simulink model "whirlybird_sim"  (Simulink 8.3)
settings: Solver=ode45  StartTime=0.0  StopTime=100  RelTol=1e-3
settings Model: Creator=Administrator  LastModifiedBy=jhl48
settings OptimizationCC: ExpressionDepthLimit=2147483647
settings DebuggingCC: FcnCallInpInsideContextMsg=UseLocalSettings

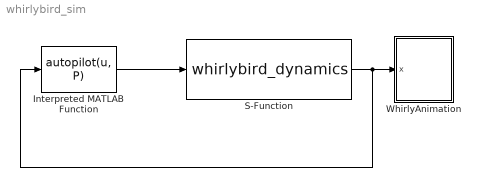
== system whirlybird_sim ==
  Interpreted MATLAB Function : MATLABFcn  MATLABFcn=autopilot(u, P)  OutputDimensions=2
  S-Function : S-Function  FunctionName=whirlybird_dynamics  Parameters=P  EnableBusSupport=off
  WhirlyAnimation : Subsystem
      mask Display: image(imread('tv.jpg'))
  wires:
  S-Function/1 -> Interpreted MATLAB Function/1, WhirlyAnimation/1(x)
  Interpreted MATLAB Function/1 -> S-Function/1

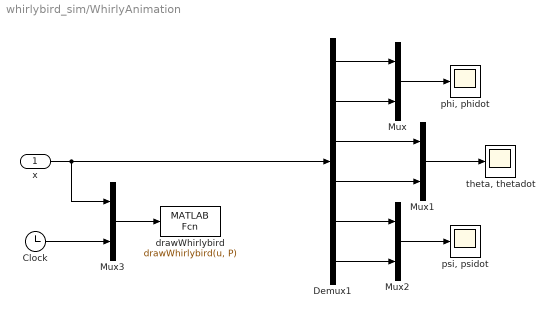
== system whirlybird_sim/WhirlyAnimation ==
  x : Inport
  Clock : Clock
  Demux1 : Demux  Outputs=6
  Mux{,1..3} (4 alike) : Mux  Inputs=2
  drawWhirlybird : MATLABFcn  MATLABFcn=drawWhirlybird(u, P)  OutputDimensions=0  SampleTime=0.1
  "phi, phidot" : Scope
      settings: TimeRange=40  YMin=-10  YMax=15  SaveName=ScopeData4
  "psi, psidot" : Scope
      settings: TimeRange=40  YMin=-2  YMax=1  SaveName=ScopeData3
  "theta, thetadot" : Scope
      settings: TimeRange=40  YMin=-2  YMax=1  SaveName=ScopeData2
  wires:
  Demux1/1 -> Mux/1
  Demux1/2 -> Mux/2
  Demux1/3 -> Mux1/1
  Demux1/4 -> Mux1/2
  Demux1/5 -> Mux2/1
  Demux1/6 -> Mux2/2
  Mux2/1 -> "psi, psidot"/1
  Mux1/1 -> "theta, thetadot"/1
  Mux/1 -> "phi, phidot"/1
  x/1 -> Mux3/1, Demux1/1
  Clock/1 -> Mux3/2
  Mux3/1 -> drawWhirlybird/1
